simulink model "hw_Loadcell_TemplateNEW"  (R2020b)
settings: Solver=FixedStepAuto  StartTime=0.0  StopTime=inf  RelTol=1e-3  EnableMultiTasking=on
libraries: simulink x7, arduinolib x7, svdutilitieslib x1
settings Model: SILPILModeSetting=veronly  EnablePacing=on  ExtModeTrigDuration=2  Creator=IDE-Admin  LastModifiedBy=helve
settings OptimizationCC: EnhancedBackFolding=on  PassReuseOutputArgsAs=Individual arguments  ZeroExternalMemoryAtStartup=off  ZeroInternalMemoryAtStartup=off  MaxStackSize=64  OptimizeBlockOrder=speed  DifferentSizesBufferReuse=on  OptimizationCustomize=off  EfficientTunableParamExpr=on
settings DebuggingCC: ParameterTunabilityLossMsg=error
settings HardwareCC: ProdBitPerPointer=32  ProdBitPerSizeT=32  ProdBitPerPtrDiffT=32  ProdLargestAtomicInteger=Long  ProdLargestAtomicFloat=Double  ProdWordSize=32  ProdHWDeviceType=ARM Compatible->ARM Cortex
settings SFSimCC: MATLABDynamicMemAlloc=off
settings RTWCC: Description=Embedded Coder  SystemTargetFile=ert.tlc  HardwareBoard=Arduino Nano 33 IoT  TemplateMakefile=ert_default_tmf  Toolchain=Arduino ARM  BuildConfiguration=Faster Runs
settings CodeAppCC: ForceParamTrailComments=on  IgnoreCustomStorageClasses=off  OperatorAnnotations=on  SimulinkDataObjDesc=on  SFDataObjDesc=on  InsertBlockDesc=on
settings ERTTargetCC: SupportContinuousTime=on  SupportVariableSizeSignals=on  ExtModeTransport=3  ExtModeStaticAllocSize=8192  ExtModeMexFile=ext_xcp  ExtModeIntrfLevel=Level2 - Open

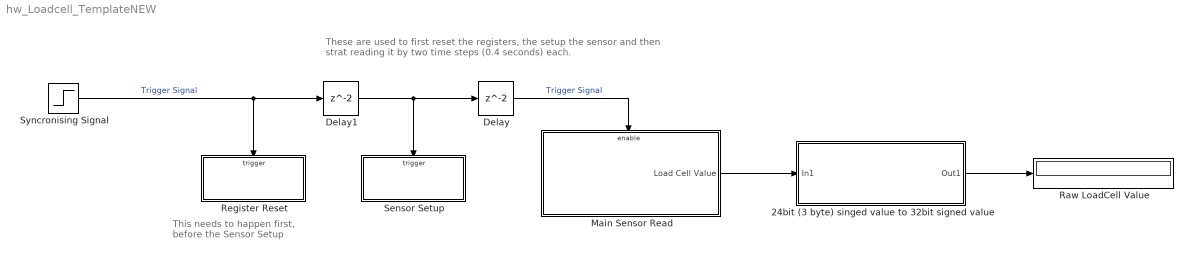
== system hw_Loadcell_TemplateNEW ==
  note: This needs to happen first,
      | before the Sensor Setup
  note: These are used to first reset the registers, the setup the sensor and
      | then strat reading it by two time steps (0.4 seconds) each.
  24bit (3 byte) singed value to 32bit signed value : Subsystem
  Delay : Delay
  Delay1 : Delay
  Main Sensor Read : Subsystem  TreatAsAtomicUnit=on
  Raw LoadCell Value : Display
      settings: Format=decimal (Stored Integer)
  Register Reset : Subsystem  TreatAsAtomicUnit=on
  Sensor Setup : Subsystem  TreatAsAtomicUnit=on
  Syncronising Signal : Step
  wires:
  Syncronising Signal/1 -> Register Reset/Trigger, Delay1/1  "Trigger Signal"
  Delay1/1 -> Sensor Setup/Trigger, Delay/1
  Delay/1 -> Main Sensor Read/Enable  "Trigger Signal"
  Main Sensor Read/1(Load Cell Value) -> 24bit (3 byte) singed value to 32bit signed value/1(In1)
  24bit (3 byte) singed value to 32bit signed value/1(Out1) -> Raw LoadCell Value/1

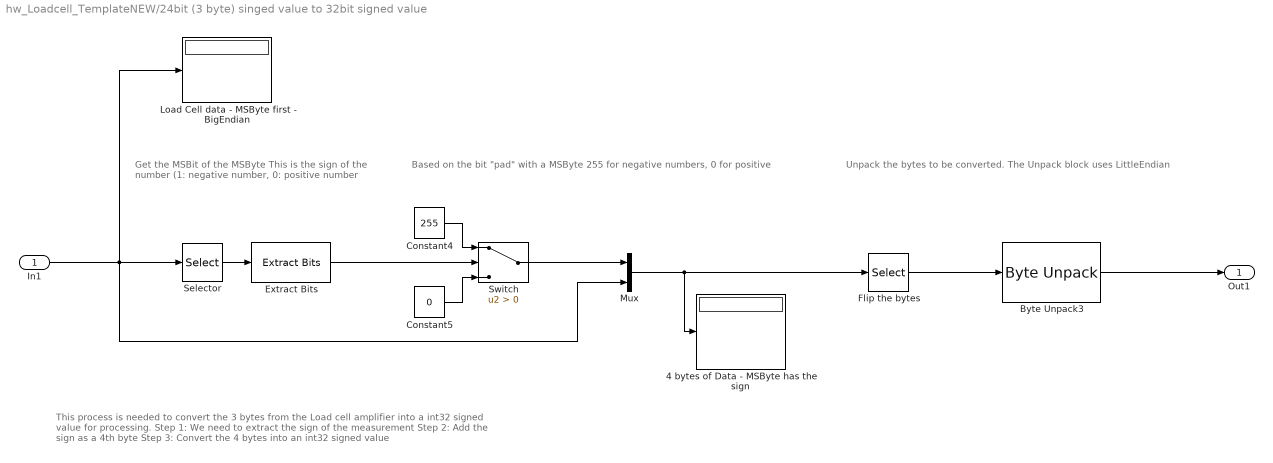
== system hw_Loadcell_TemplateNEW/24bit (3 byte) singed value to 32bit signed value ==
  note: Unpack the bytes to be converted.
      | The Unpack block uses LittleEndian
  note: This process is needed to convert the 3 bytes from the Load cell amplifier into a int32 signed value for processing.
      | Step 1: We need to extract the sign of the measurement
      | Step 2: Add the sign as a 4th byte
      | Step 3: Convert the 4 bytes into an int32 signed value
  note: Based on the bit "pad" with a MSByte
      | 255 for negative numbers, 0 for positive
  note: Get the MSBit of the MSByte
      | This is the sign of the number
      | (1: negative number, 0: positive number
  In1 : Inport
  4 bytes of Data - MSByte has the sign : Display
  Byte Unpack3 : svdutilitieslib/Byte Unpack  dimensions={[1]}  datatypes={'int32'}  byteAlign=1  blockPlatform=arduinoert
      settings: SourceProductBaseCode=ANDROID,ARDUINO,ML_ARDUINO,ECCORTEXA,ECCORTEXR,SC_BEAGLEBONE_BLUE,EC_FREEDOM_BOARD,EC_FRDM_K64F,INTEL_BLOCKSET,JETSONCPU,MICROBIT,NUCLEO,NVIDIA,PX4AUTOPILOTS,RASPPIIO,STMICRODIS,TIC2000,XILINX_BLOCKSET
  Constant4 : Constant  Value=255  OutDataTypeStr=uint8  SampleTime=-1
  Constant5 : Constant  Value=0  OutDataTypeStr=uint8  SampleTime=-1
  Extract Bits : simulink/Logic and Bit Operations/Extract Bits  bitsToExtract=Range of bits  numBits=8  bitIdxRange=[7]  outScalingMode=Preserve fixed-point scaling
  Flip the bytes : Selector  InputPortWidth=4  IndexOptions=Index vector (dialog)  Indices=[4 3 2 1]  OutputSizes=1
  Load Cell data - MSByte first - BigEndian : Display
  Mux : Mux  Inputs=2
  Selector : Selector  InputPortWidth=3  IndexOptions=Index vector (dialog)  Indices=[1]  OutputSizes=1
  Switch : Switch  Criteria=u2 > Threshold
  Out1 : Outport
  wires:
  In1/1 -> Selector/1, Mux/2, Load Cell data - MSByte first - BigEndian/1
  Flip the bytes/1 -> Byte Unpack3/1
  Selector/1 -> Extract Bits/1
  Extract Bits/1 -> Switch/2
  Constant5/1 -> Switch/3
  Constant4/1 -> Switch/1
  Switch/1 -> Mux/1
  Mux/1 -> Flip the bytes/1, 4 bytes of Data - MSByte has the sign/1
  Byte Unpack3/1 -> Out1/1

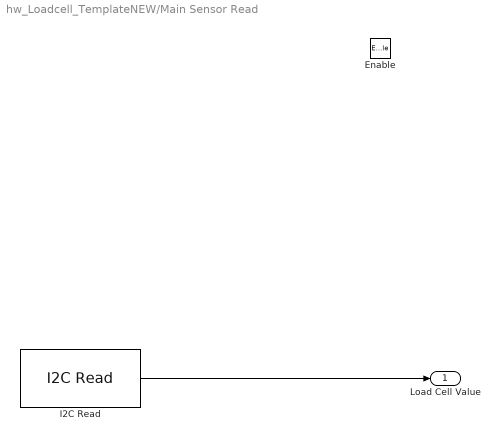
== system hw_Loadcell_TemplateNEW/Main Sensor Read ==
  Enable : EnablePort
  I2C Read : arduinolib/I2C Read  I2CModule=0  Mode=Master  SlaveAddress=0x2A  SlaveByteOrder=BigEndian  Direction=Receiver  RegisterAddressMode=on  RegisterAddress=0x12  SlaveDataType=uint8  DataLength=3  NoAck=off  RepeatedStart=off  OutputStatus=off  blockPlatform=ARDUINO  SampleTime=-1
      settings: SourceProductBaseCode=ARDUINO
      settings: AttributesFormatString=|
      | %<RegisterAddress>
      | %<SlaveDataType>
  Load Cell Value : Outport  VectorParamsAs1DForOutWhenUnconnected=off
  wires:
  I2C Read/1 -> Load Cell Value/1

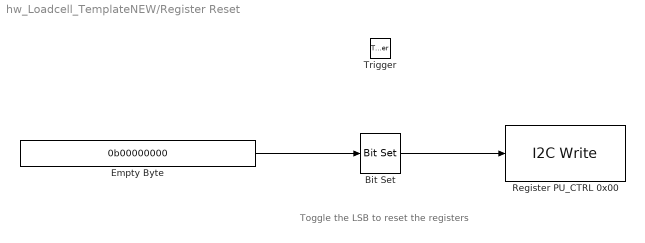
== system hw_Loadcell_TemplateNEW/Register Reset ==
  note: Toggle the LSB to reset the registers
  Trigger : TriggerPort  VariantControl=Variant
  Bit Set : simulink/Logic and Bit Operations/Bit Set  iBit=0
      settings: SourceProductBaseCode=SL
  Empty Byte : Constant  Value=0b00000000  OutDataTypeStr=uint8  SampleTime=-1
  Register PU_CTRL 0x00 : arduinolib/I2C Write  I2CModule=0  Mode=Master  SlaveAddress=hex2dec( '2A' )  SlaveByteOrder=BigEndian  Direction=Transmitter  RegisterAddressMode=on  RegisterAddress=hex2dec( '00' )  SlaveDataType=uint8  DataLength=1  NoAck=off  RepeatedStart=off  OutputStatus=off  blockPlatform=ARDUINO
      settings: SourceProductBaseCode=ARDUINO
      settings: AttributesFormatString=|
      | Register
      | %<RegisterAddress>
  wires:
  Bit Set/1 -> Register PU_CTRL 0x00/1
  Empty Byte/1 -> Bit Set/1

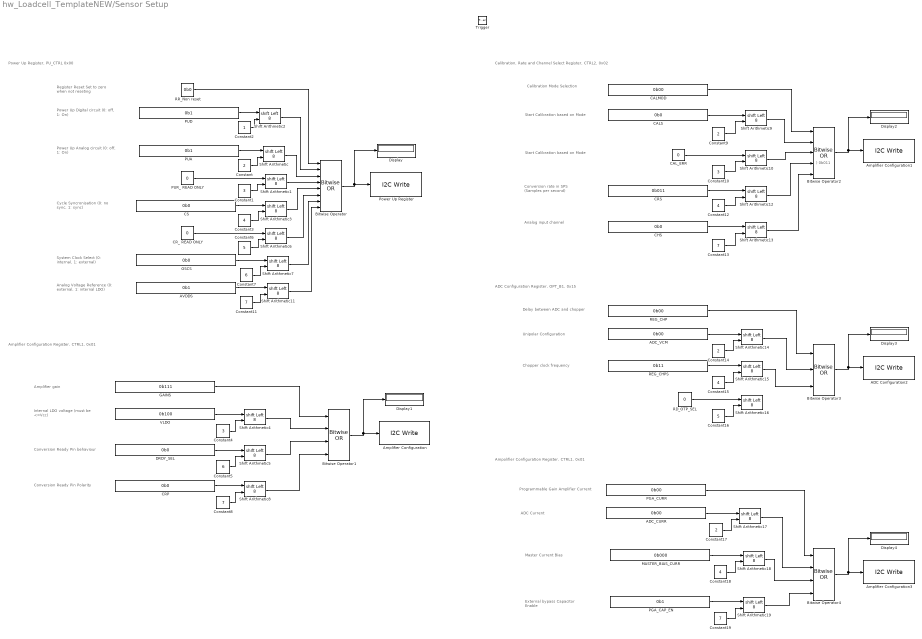
== system hw_Loadcell_TemplateNEW/Sensor Setup ==
  note: ) 0b011
  note: Power Up Digital circuit
      | (0: off, 1: On)
  note: Register Reset
      | Set to zero when not reseting
  note: Power Up Register, PU_CTRL 0x00
  note: Amplifier Configuration Register, CTRL1, 0x01
  note: Calibration, Rate and Channel Select Register, CTRL2, 0x02
  note: Power Up Analog circuit
      | (0: off, 1: On)
  note: Cycle Syncronisation
      | (0: no sync, 1: sync)
  note: System Clock Select
      | (0: internal, 1: external)
  note: Analog Voltage Reference
      | (0: external, 1: internal LDO)
  note: ADC Configuration Register, OPT_B1, 0x15
  note: Ampolifier Configuration Register, CTRL1, 0x01
  note: Amplifier gain
  note: Internal LDO voltage
      | (must be <=Vcc)
  note: Conversion Ready Pin behaviour
  note: Conversion Ready Pin Polarity
  note: Calibration Mode Selection
  note: Start Calibration based on Mode
  note: Start Calibration based on Mode
  note: Conversion rate in SPS
      | (Samples per second)
  note: Analog input channel
  note: Delay between ADC and chopper
  note: Unipolar Configuration
  note: Chopper clock frequency
  note: ADC Current
  note: Programmable Gain Amplifier Current
  note: Master Current Bias
  note: External bypass Capacitor Enable
  Trigger : TriggerPort  VariantControl=Variant
  ADC Configuration2 : arduinolib/I2C Write  Priority=1  I2CModule=0  Mode=Master  SlaveAddress=0x2A  SlaveByteOrder=BigEndian  Direction=Transmitter  RegisterAddressMode=on  RegisterAddress=0x15  SlaveDataType=uint8  DataLength=1  NoAck=off  RepeatedStart=off  OutputStatus=off  blockPlatform=ARDUINO
      settings: SourceProductBaseCode=ARDUINO
      settings: AttributesFormatString=|
      | Register
      | %<RegisterAddress>
  ADC_CURR : Constant  Value=0b00  OutDataTypeStr=uint8  SampleTime=-1
  ADC_VCM : Constant  Value=0b00  OutDataTypeStr=uint8  SampleTime=-1
  AVDDS : Constant  Value=0b1  OutDataTypeStr=uint8  SampleTime=-1
  Amplifier Configuration : arduinolib/I2C Write  Priority=1  I2CModule=0  Mode=Master  SlaveAddress=0x2A  SlaveByteOrder=BigEndian  Direction=Transmitter  RegisterAddressMode=on  RegisterAddress=0x01  SlaveDataType=uint8  DataLength=1  NoAck=off  RepeatedStart=off  OutputStatus=off  blockPlatform=ARDUINO
      settings: SourceProductBaseCode=ARDUINO
      settings: AttributesFormatString=|
      | Register
      | %<RegisterAddress>
  Amplifier Configuration1 : arduinolib/I2C Write  Priority=1  I2CModule=0  Mode=Master  SlaveAddress=0x2A  SlaveByteOrder=BigEndian  Direction=Transmitter  RegisterAddressMode=on  RegisterAddress=0x02  SlaveDataType=uint8  DataLength=1  NoAck=off  RepeatedStart=off  OutputStatus=off  blockPlatform=ARDUINO
      settings: SourceProductBaseCode=ARDUINO
      settings: AttributesFormatString=|
      | Register
      | %<RegisterAddress>
  Amplifier Configuration3 : arduinolib/I2C Write  Priority=1  I2CModule=0  Mode=Master  SlaveAddress=0x2A  SlaveByteOrder=BigEndian  Direction=Transmitter  RegisterAddressMode=on  RegisterAddress=0x1C  SlaveDataType=uint8  DataLength=1  NoAck=off  RepeatedStart=off  OutputStatus=off  blockPlatform=ARDUINO
      settings: SourceProductBaseCode=ARDUINO
      settings: AttributesFormatString=|
      | Register
      | %<RegisterAddress>
  Bitwise Operator : simulink/Logic and Bit Operations/Bitwise Operator  logicop=OR  UseBitMask=off  NumInputPorts=8  BitMask=bin2dec('11011001')  BitMaskRealWorld=Stored Integer
  Bitwise Operator1 : simulink/Logic and Bit Operations/Bitwise Operator  logicop=OR  UseBitMask=off  NumInputPorts=4  BitMask=bin2dec('11011001')  BitMaskRealWorld=Stored Integer
  Bitwise Operator2 : simulink/Logic and Bit Operations/Bitwise Operator  logicop=OR  UseBitMask=off  NumInputPorts=5  BitMask=bin2dec('11011001')  BitMaskRealWorld=Stored Integer
  Bitwise Operator3 : simulink/Logic and Bit Operations/Bitwise Operator  logicop=OR  UseBitMask=off  NumInputPorts=3  BitMask=bin2dec('11011001')  BitMaskRealWorld=Stored Integer
  Bitwise Operator4 : simulink/Logic and Bit Operations/Bitwise Operator  logicop=OR  UseBitMask=off  NumInputPorts=4  BitMask=bin2dec('11011001')  BitMaskRealWorld=Stored Integer
  CALMOD : Constant  Value=0b00  OutDataTypeStr=uint8  SampleTime=-1
  CALS : Constant  Value=0b0  OutDataTypeStr=uint8  SampleTime=-1
  CAL_ERR : Constant  Value=0  OutDataTypeStr=uint8  SampleTime=-1
  CHS : Constant  Value=0b0  OutDataTypeStr=uint8  SampleTime=-1
  CRP : Constant  Value=0b0  OutDataTypeStr=uint8  SampleTime=-1
  CRS : Constant  Value=0b011  OutDataTypeStr=uint8  SampleTime=-1
  CR_ READ ONLY : Constant  Value=0  OutDataTypeStr=uint8  SampleTime=-1
  "CS " : Constant  Value=0b0  OutDataTypeStr=uint8  SampleTime=-1
  Constant : Constant  Value=2  OutDataTypeStr=uint8  SampleTime=-1
  Constant1 : Constant  Value=3  OutDataTypeStr=uint16  SampleTime=-1
  Constant10 : Constant  Value=3  OutDataTypeStr=uint16  SampleTime=-1
  Constant{8,11,13,19} (4 alike) : Constant  Value=7  OutDataTypeStr=uint16  SampleTime=-1
  Constant{3,12,15,18} (4 alike) : Constant  Value=4  OutDataTypeStr=uint16  SampleTime=-1
  Constant14 : Constant  Value=2  OutDataTypeStr=uint16  SampleTime=-1
  Constant16 : Constant  Value=5  OutDataTypeStr=uint16  SampleTime=-1
  Constant17 : Constant  Value=2  OutDataTypeStr=uint16  SampleTime=-1
  Constant2 : Constant  OutDataTypeStr=uint8  SampleTime=-1
  Constant4 : Constant  Value=3  OutDataTypeStr=uint16  SampleTime=-1
  Constant5 : Constant  Value=6  OutDataTypeStr=uint16  SampleTime=-1
  Constant6 : Constant  Value=5  OutDataTypeStr=uint16  SampleTime=-1
  Constant7 : Constant  Value=6  OutDataTypeStr=uint16  SampleTime=-1
  Constant9 : Constant  Value=2  OutDataTypeStr=uint16  SampleTime=-1
  DRDY_SEL : Constant  Value=0b0  OutDataTypeStr=uint8  SampleTime=-1
  Display{,1..4} (5 alike) : Display
      settings: Format=hex (Stored Integer)
  GAINS : Constant  Value=0b111  OutDataTypeStr=uint8  SampleTime=-1
  MASTER_BIAS_CURR : Constant  Value=0b000  OutDataTypeStr=uint8  SampleTime=-1
  OSCS : Constant  Value=0b0  OutDataTypeStr=uint8  SampleTime=-1
  PGA_CAP_EN : Constant  Value=0b1  OutDataTypeStr=uint8  SampleTime=-1
  PGA_CURR : Constant  Value=0b00  OutDataTypeStr=uint8  SampleTime=-1
  PUA : Constant  Value=0b1  OutDataTypeStr=uint8  SampleTime=-1
  PUD : Constant  Value=0b1  OutDataTypeStr=uint8  SampleTime=-1
  PUR_ READ ONLY : Constant  Value=0  OutDataTypeStr=uint8  SampleTime=-1
  Power Up Register : arduinolib/I2C Write  Priority=1  I2CModule=0  Mode=Master  SlaveAddress=hex2dec( '2A' )  SlaveByteOrder=BigEndian  Direction=Transmitter  RegisterAddressMode=on  RegisterAddress=0x00  SlaveDataType=uint8  DataLength=1  NoAck=off  RepeatedStart=off  OutputStatus=off  blockPlatform=ARDUINO
      settings: SourceProductBaseCode=ARDUINO
      settings: AttributesFormatString=|
      | Register
      | %<RegisterAddress>
  RD_OTP_SEL : Constant  Value=0  OutDataTypeStr=uint8  SampleTime=-1
  REG_CHP : Constant  Value=0b00  OutDataTypeStr=uint8  SampleTime=-1
  REG_CHPS : Constant  Value=0b11  OutDataTypeStr=uint8  SampleTime=-1
  RR_Non reset : Constant  Value=0b0  OutDataTypeStr=uint8  SampleTime=-1
  Shift Arithmetic{,1..19} (20 alike) : ArithShift  BitShiftNumberSource=Input port  BitShiftNumber=8  BitShiftDirection=Left
      settings: InputPortMap=u0,p1
  VLDO : Constant  Value=0b100  OutDataTypeStr=uint8  SampleTime=-1
  wires:
  Constant/1 -> Shift Arithmetic/2
  Constant1/1 -> Shift Arithmetic1/2
  PUA/1 -> Shift Arithmetic/1
  Bitwise Operator/1 -> Display/1, Power Up Register/1
  RR_Non reset/1 -> Bitwise Operator/1
  Constant2/1 -> Shift Arithmetic2/2
  PUD/1 -> Shift Arithmetic2/1
  Shift Arithmetic2/1 -> Bitwise Operator/2
  Shift Arithmetic/1 -> Bitwise Operator/3
  PUR_ READ ONLY/1 -> Shift Arithmetic1/1
  Shift Arithmetic1/1 -> Bitwise Operator/4
  "CS "/1 -> Shift Arithmetic3/1
  Constant3/1 -> Shift Arithmetic3/2
  Shift Arithmetic3/1 -> Bitwise Operator/5
  Constant6/1 -> Shift Arithmetic6/2
  CR_ READ ONLY/1 -> Shift Arithmetic6/1
  Shift Arithmetic6/1 -> Bitwise Operator/6
  Constant7/1 -> Shift Arithmetic7/2
  Constant11/1 -> Shift Arithmetic11/2
  OSCS/1 -> Shift Arithmetic7/1
  Shift Arithmetic7/1 -> Bitwise Operator/7
  AVDDS/1 -> Shift Arithmetic11/1
  Shift Arithmetic11/1 -> Bitwise Operator/8
  Bitwise Operator1/1 -> Amplifier Configuration/1, Display1/1
  GAINS/1 -> Bitwise Operator1/1
  VLDO/1 -> Shift Arithmetic4/1
  Shift Arithmetic4/1 -> Bitwise Operator1/2
  Constant4/1 -> Shift Arithmetic4/2
  DRDY_SEL/1 -> Shift Arithmetic5/1
  Constant5/1 -> Shift Arithmetic5/2
  Shift Arithmetic5/1 -> Bitwise Operator1/3
  Shift Arithmetic8/1 -> Bitwise Operator1/4
  Constant8/1 -> Shift Arithmetic8/2
  CRP/1 -> Shift Arithmetic8/1
  Bitwise Operator2/1 -> Amplifier Configuration1/1, Display2/1
  Bitwise Operator3/1 -> ADC Configuration2/1, Display3/1
  Bitwise Operator4/1 -> Amplifier Configuration3/1, Display4/1
  CALMOD/1 -> Bitwise Operator2/1
  CALS/1 -> Shift Arithmetic9/1
  Shift Arithmetic9/1 -> Bitwise Operator2/2
  Constant9/1 -> Shift Arithmetic9/2
  CAL_ERR/1 -> Shift Arithmetic10/1
  Constant10/1 -> Shift Arithmetic10/2
  Shift Arithmetic10/1 -> Bitwise Operator2/3
  Constant12/1 -> Shift Arithmetic12/2
  CRS/1 -> Shift Arithmetic12/1
  Shift Arithmetic12/1 -> Bitwise Operator2/4
  CHS/1 -> Shift Arithmetic13/1
  Shift Arithmetic13/1 -> Bitwise Operator2/5
  Constant13/1 -> Shift Arithmetic13/2
  REG_CHP/1 -> Bitwise Operator3/1
  ADC_VCM/1 -> Shift Arithmetic14/1
  Constant14/1 -> Shift Arithmetic14/2
  Shift Arithmetic14/1 -> Bitwise Operator3/2
  REG_CHPS/1 -> Shift Arithmetic15/1
  Constant15/1 -> Shift Arithmetic15/2
  Shift Arithmetic15/1 -> Bitwise Operator3/3
  Constant16/1 -> Shift Arithmetic16/2
  RD_OTP_SEL/1 -> Shift Arithmetic16/1
  PGA_CURR/1 -> Bitwise Operator4/1
  ADC_CURR/1 -> Shift Arithmetic17/1
  Shift Arithmetic17/1 -> Bitwise Operator4/2
  Constant17/1 -> Shift Arithmetic17/2
  Shift Arithmetic18/1 -> Bitwise Operator4/3
  MASTER_BIAS_CURR/1 -> Shift Arithmetic18/1
  Constant18/1 -> Shift Arithmetic18/2
  PGA_CAP_EN/1 -> Shift Arithmetic19/1
  Shift Arithmetic19/1 -> Bitwise Operator4/4
  Constant19/1 -> Shift Arithmetic19/2
